simulink model "SuspensionSystem"  (R2025a)
settings: Solver=VariableStepAuto  StartTime=0.0  StopTime=10  RelTol=1e-3
undefined symbols (not defined in the file): cs, ks, mass_payload, mass_robot
settings Model: DataDictionary=Constants.sldd  Creator=yaremadzulynsky  LastModifiedBy=levirogalla

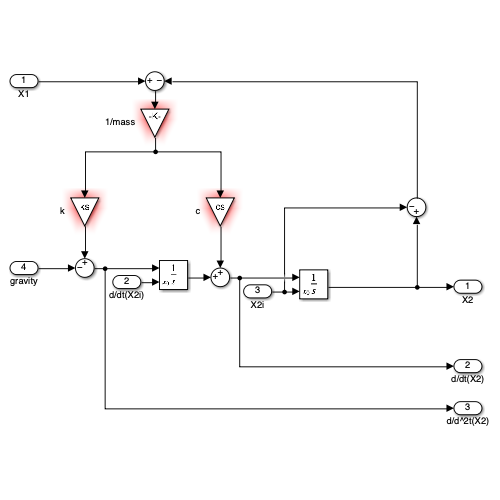
[thumbnail: Simulink's stored preview of the top-level diagram]
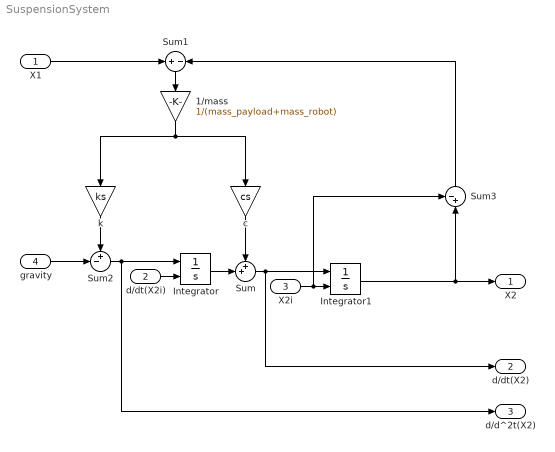
== system SuspensionSystem ==
  X1 : Inport
  d/dt(X2i) : Inport  Port=2
  X2i : Inport  Port=3
  gravity : Inport  Port=4
  1/mass : Gain  Gain=1/(mass_payload+mass_robot)
  Integrator : Integrator  InitialConditionSource=external
  Integrator1 : Integrator  InitialConditionSource=external
  Sum : Sum  Inputs=++|
  Sum1 : Sum  Inputs=+-
  Sum2 : Sum  Inputs=+-|
  Sum3 : Sum  Inputs=-+|
  c : Gain  Gain=cs
  k : Gain  Gain=ks
  X2 : Outport
  d/dt(X2) : Outport  Port=2
  d/d^2t(X2) : Outport  Port=3
  wires:
  Integrator/1 -> Sum/2
  Sum2/1 -> d/d^2t(X2)/1, Integrator/1
  X1/1 -> Sum1/1
  gravity/1 -> Sum2/2
  Integrator1/1 -> Sum3/2, X2/1
  Sum1/1 -> 1/mass/1
  Sum/1 -> d/dt(X2)/1, Integrator1/1
  d/dt(X2i)/1 -> Integrator/2
  c/1 -> Sum/1
  k/1 -> Sum2/1
  X2i/1 -> Sum3/1, Integrator1/2
  1/mass/1 -> k/1, c/1
  Sum3/1 -> Sum1/2
